simulink model "OpenLoop"  (R2025b)
settings: Solver=FixedStepAuto  StartTime=0.0  StopTime=10  FixedStep=0.001  RelTol=1e-3
settings Model: Creator=mj  LastModifiedBy=mj

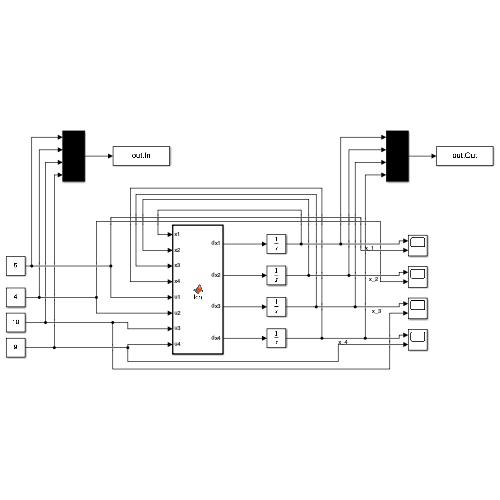
[thumbnail: Simulink's stored preview of the top-level diagram]
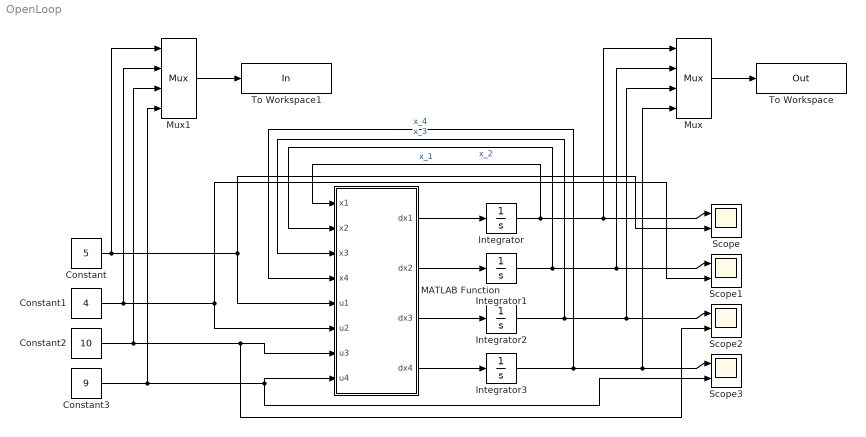
== system OpenLoop ==
  Constant : Constant  Value=5
  Constant1 : Constant  Value=4
  Constant2 : Constant  Value=10
  Constant3 : Constant  Value=9
  Integrator : Integrator  InitialCondition=10
  Integrator1 : Integrator  InitialCondition=9
  Integrator2 : Integrator  InitialCondition=6
  Integrator3 : Integrator  InitialCondition=5
  MATLAB Function : MATLAB Function  TreatAsAtomicUnit=on
  Mux : Mux
  Mux1 : Mux
  Scope{,1..3} (4 alike) : Scope  NumInputPorts=2
      Scope settings: ActiveDisplayYMinimum=3.8645263574238582  ActiveDisplayYMaximum=15.219262783185282
      Scope1 settings: ActiveDisplayYMinimum=-18.368026813774154  ActiveDisplayYMaximum=18.139471063576107
      Scope2 settings: ActiveDisplayYMinimum=-16.844418920799139  ActiveDisplayYMaximum=17.491280096998292  DataLoggingVariableName=ScopeData2
      Scope3 settings: ActiveDisplayYMinimum=-5.7161497380140025  ActiveDisplayYMaximum=10.635127748668223  DataLoggingVariableName=ScopeData3
  To Workspace : ToWorkspace  VariableName=Out  SaveFormat=Timeseries  SampleTime=-1
  To Workspace1 : ToWorkspace  VariableName=In  SaveFormat=Timeseries  SampleTime=-1
  wires:
  MATLAB Function/1(dx1) -> Integrator/1
  MATLAB Function/4(dx4) -> Integrator3/1
  MATLAB Function/3(dx3) -> Integrator2/1
  MATLAB Function/2(dx2) -> Integrator1/1
  Integrator/1 -> Mux/1, Scope/1, MATLAB Function/1(x1)  "x_1"
  Integrator1/1 -> Mux/2, Scope1/1, MATLAB Function/2(x2)  "x_2"
  Integrator2/1 -> Mux/3, Scope2/1, MATLAB Function/3(x3)  "x_3"
  Integrator3/1 -> Mux/4, Scope3/1, MATLAB Function/4(x4)  "x_4"
  Constant/1 -> MATLAB Function/5(u1), Scope/2, Mux1/1
  Constant3/1 -> Mux1/4, Scope3/2, MATLAB Function/8(u4)
  Constant2/1 -> Mux1/3, Scope2/2, MATLAB Function/7(u3)
  Constant1/1 -> MATLAB Function/6(u2), Scope1/2, Mux1/2
  Mux/1 -> To Workspace/1
  Mux1/1 -> To Workspace1/1

== matlab function OpenLoop/MATLAB Function ==
  data: x1 input; dx1 output; x2 input; x3 input; x4 input; u1 input; u2 input; u3 input; u4 input; dx2 output; dx3 output; dx4 output
function [dx1,dx2,dx3,dx4] = fcn(x1,x2,x3,x4,u1,u2,u3,u4)
L1 = 557.7;
L2 = 1016.9;
L3 = 41.0;
L4 = -628.9;

M11 = -86.1;
M22 = -392.4;
M23 = 263.9;
M32 = -218.3;
M33 = -7.6;
M41 = 43.4;
M44 = -113.5;

N111 = 1.8;
N121 = -2.2;
N131 = -2.3;
N141 = -6.8;
N212 = 75.0;
N313 = 5.0;
N314 = 3.9;
N414 = 2.9;
N424 = -9.8;
N434 = 6.3;
N444 = -7.3;

O2222 = -2.5;
O2233 = -2.5;
O3223 = -0.2;
O3333 = -0.2;

dx1 = L1 + M11*x1 + N111*x1^2 + N121*x1*x2 + N131*x1*x3 + N141*x1*x4 + u1;
dx2 = L2 + M22*x2 + M23*x3 + N212*x1*x2 + O2222*x2^3 + O2233*x2*x3^2 + u2;
dx3 = L3 + M32*x2 + M33*x3 + N313*x1*x3 + N314*x1*x4 + O3223*x3*x2^2 + O3333*x3^3 + u3;
dx4 = L4 + M41*x1 + M44*x4 + N414*x1*x4 + N424*x2*x4 + N434*x3*x4 + N444*x4^2 + u4;
